simulink model "MASH"  (R2013b)
settings: Solver=FixedStepDiscrete  StartTime=0.0  StopTime=1.0  RelTol=1e-3
values from neighbouring files (symbols this model uses):
  ftest = 9e6    (= 9000000)    [Model.m]
  nLev = 512    [Model.m]
  Ts = 1/Fs    (= 2.03450520833e-09)    [Model.m]
libraries: dspsrcs4 x1
settings Model: Creator=o_cotte  LastModifiedBy=o_cotte
settings DataIOCC: LimitDataPoints=off  SaveFormat=Dataset
settings OptimizationCC: LifeSpan=auto  SimCompilerOptimization=off
settings DebuggingCC: UnderspecifiedInitializationDetection=Simplified  MergeDetectMultiDrivingBlocksExec=error  SolverPrmCheckMsg=none  FcnCallInpInsideContextMsg=error  FrameProcessingCompatibilityMsg=error  SFUnexpectedBacktrackingDiag=error  SFNoUnconditionalDefaultTransitionDiag=error
settings HardwareCC: ProdBitPerPointer=64  ProdLargestAtomicFloat=Float  ProdIntDivRoundTo=Zero  ProdEndianess=LittleEndian  ProdWordSize=64  ProdHWDeviceType=Intel->x86-64 (Windows64)
settings ModelReferenceCC: PropagateSignalLabelsOutOfModel=on
settings RTWCC: RTWCompilerOptimization=off
settings GRTTargetCC: CodeReplacementLibrary=None  GeneratePreprocessorConditionals=Use local settings  CPPClassGenCompliant=on

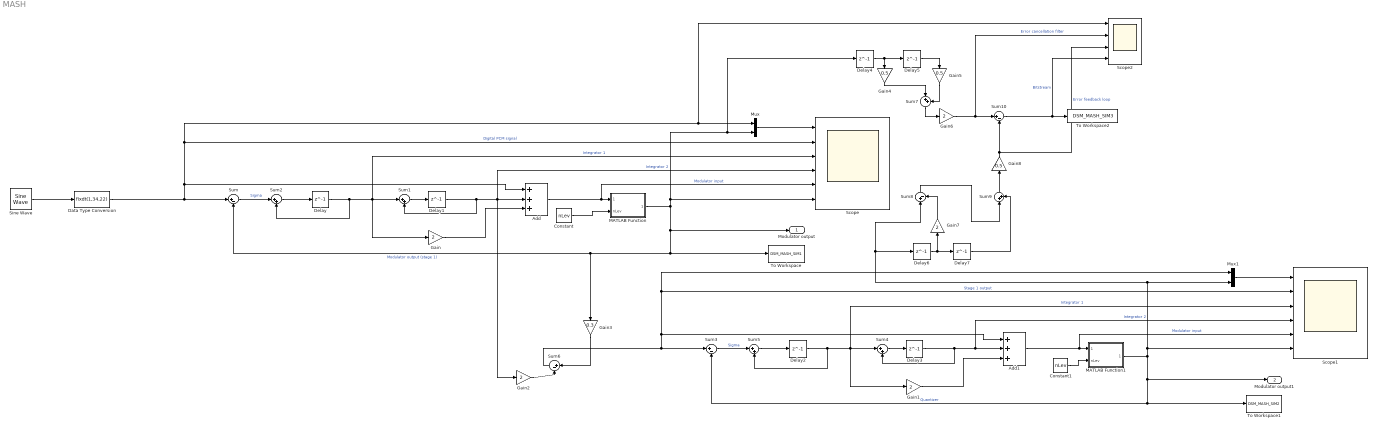
== system MASH ==
  Add : Sum  Inputs=+++  OutDataTypeStr=Inherit: Same as accumulator  LockScale=on
  Add1 : Sum  Inputs=+++  OutDataTypeStr=fixdt(1,34,23)
  Constant : Constant  Value=nLev
  Constant1 : Constant  Value=nLev
  Data Type Conversion : DataTypeConversion  OutDataTypeStr=fixdt(1,34,22)  LockScale=on
  Delay{,1..7} (8 alike) : Delay  DelayLength=1  InitialCondition=0
  Gain : Gain  Gain=2  OutDataTypeStr=Inherit: Same as input  LockScale=on
  Gain1 : Gain  Gain=2  OutDataTypeStr=fixdt(1,34,23)
  Gain2 : Gain  Gain=2  OutDataTypeStr=fixdt(1,34,23)
  Gain3 : Gain  Gain=0.3  OutDataTypeStr=Inherit: Same as input  LockScale=on
  Gain4 : Gain  Gain=0.5  OutDataTypeStr=Inherit: Same as input  ParamDataTypeStr=Inherit: Same as input  LockScale=on
  Gain5 : Gain  Gain=0.5  OutDataTypeStr=Inherit: Same as input  ParamDataTypeStr=Inherit: Same as input  LockScale=on
  Gain6 : Gain  Gain=2  OutDataTypeStr=Inherit: Same as input  LockScale=on
  Gain7 : Gain  Gain=2  OutDataTypeStr=fixdt(1,34,23)
  Gain8 : Gain  Gain=0.5  OutDataTypeStr=Inherit: Same as input  ParamDataTypeStr=Inherit: Same as input  LockScale=on
  MATLAB Function : MATLAB Function  TreatAsAtomicUnit=on
  MATLAB Function1 : MATLAB Function  TreatAsAtomicUnit=on
  Mux : Mux  Inputs=2
  Mux1 : Mux  Inputs=2
  Scope : Scope  NumInputPorts=6
  Scope1 : Scope  NumInputPorts=6
  Scope2 : Scope  NumInputPorts=4
  Sine Wave : dspsrcs4/Sine Wave  Amplitude=1  Frequency=ftest  Phase=0  SampleMode=Discrete  OutComplex=Real  CompMethod=Trigonometric fcn  TableSize=Speed  SampleTime=Ts  SamplesPerFrame=1  ResetState=Restart at time zero  dataType=double  wordLen=16  udDataType=sfix(16)  fracBitsMode=Best precision  numFracBits=15  OutDataTypeStr=double  LastOutDataTypeStr=double
  Sum{,3,6,8,10} (5 alike) : Sum  Inputs=|+-  OutDataTypeStr=Inherit: Same as accumulator  LockScale=on
  Sum{1..2,7,9} (4 alike) : Sum  Inputs=|++  OutDataTypeStr=Inherit: Same as accumulator  LockScale=on
  Sum4 : Sum  Inputs=|++  OutDataTypeStr=fixdt(1,34,23)
  Sum5 : Sum  Inputs=|++  OutDataTypeStr=fixdt(1,34,23)
  To Workspace : ToWorkspace  VariableName=DSM_MASH_SIM1  SampleTime=-1
  To Workspace1 : ToWorkspace  VariableName=DSM_MASH_SIM2  SampleTime=-1
  To Workspace2 : ToWorkspace  VariableName=DSM_MASH_SIM3  SampleTime=-1
  Modulator output : Outport
  Modulator output1 : Outport  Port=2
  wires:
  Gain5/1 -> Sum7/2
  Gain/1 -> Add/3
  Delay2/1 -> Sum5/2, Sum4/1, Scope1/3, Gain1/1  "Integrator 1"
  Mux/1 -> Scope/1
  Delay7/1 -> Sum9/2
  Delay1/1 -> Sum1/2, Gain2/1, Scope/4, Add/2  "Integrator 2"
  Sum3/1 -> Sum5/1  "Sigma"
  Delay5/1 -> Gain5/1
  Mux1/1 -> Scope1/1
  Add1/1 -> MATLAB Function1/1(quant_in), Scope1/5  "Modulator input"
  MATLAB Function1/1(quant_out) -> Scope1/6, Sum8/1, Delay6/1, Mux1/2, Modulator output1/1, Sum3/2, To Workspace1/1  "Quantizer"
  Gain7/1 -> Sum8/2
  Delay4/1 -> Delay5/1, Gain4/1
  Sum9/1 -> Gain8/1
  Constant/1 -> MATLAB Function/2(nLev)
  Data Type Conversion/1 -> Sum/1, Scope/2, Scope2/1, Mux/1, Add/1  "Digital PCM signal"
  Sum4/1 -> Delay3/1
  Add/1 -> Scope/5, MATLAB Function/1(quant_in)  "Modulator input"
  Sum6/1 -> Sum3/1, Scope1/2, Mux1/1, Add1/1  "Stage 1 output"
  Sum2/1 -> Delay/1
  Sum/1 -> Sum2/1  "Sigma"
  Gain3/1 -> Sum6/1
  Delay/1 -> Sum2/2, Sum1/1, Scope/3, Gain/1  "Integrator 1"
  Gain6/1 -> Sum10/1, Scope2/2  "Error cancellation filter"
  Gain2/1 -> Sum6/2
  Sum8/1 -> Sum9/1
  Gain1/1 -> Add1/3
  Sum10/1 -> Scope2/4, To Workspace2/1  "Bitstream"
  Sine Wave/1 -> Data Type Conversion/1
  Delay6/1 -> Gain7/1, Delay7/1
  Constant1/1 -> MATLAB Function1/2(nLev)
  Delay3/1 -> Sum4/2, Scope1/4, Add1/2  "Integrator 2"
  Gain4/1 -> Sum7/1
  Sum7/1 -> Gain6/1
  Sum5/1 -> Delay2/1
  Gain8/1 -> Scope2/3, Sum10/2  "Error feedback loop"
  MATLAB Function/1(quant_out) -> Scope/6, Delay4/1, Mux/2, Modulator output/1, Gain3/1, Sum/2, To Workspace/1  "Modulator output (stage 1)"
  Sum1/1 -> Delay1/1

== matlab function MASH/MATLAB Function ==
  data: quant_in input; quant_out output; nLev input
function quant_out = fcn(quant_in,nLev)
%#codegen
% if u < 0
%     y = fi(-1,1,34,23);
% else
%     y = fi(1,1,34,23);
% end
% nLev=512;
st=fi(nLev-2,1,34,22);
quant_out=fi(0,1,34,22);
if quant_in < -st
    quant_out = fi(-nLev+1,1,34,22);
    %     return;
elseif quant_in >= st
    quant_out = fi(nLev-1,1,34,22);
    %     return;
else
    for n=1:nLev-2
        k=fi(n,1,34,22);
        if quant_in >= -nLev + 2*k && quant_in < -nLev + 2*(k+1)
            quant_out = fi(2*k-1-nLev,1,34,22);
        end
    end
end

== matlab function MASH/MATLAB Function1 ==
  data: quant_in input; quant_out output; nLev input
function quant_out = fcn(quant_in,nLev)
%#codegen
% if u < 0
%     y = fi(-1,1,34,23);
% else
%     y = fi(1,1,34,23);
% end
% nLev=512;
st=fi(nLev-2,1,34,22);
quant_out=fi(0,1,34,22);
if quant_in < -st
    quant_out = fi(-nLev+1,1,34,22);
    %     return;
elseif quant_in >= st
    quant_out = fi(nLev-1,1,34,22);
    %     return;
else
    for n=1:nLev-2
        k=fi(n,1,34,22);
        if quant_in >= -nLev + 2*k && quant_in < -nLev + 2*(k+1)
            quant_out = fi(2*k-1-nLev,1,34,22);
        end
    end
end

== matlab function MASH/MATLAB Function1 ==
  data: quant_in input; quant_out output; nLev input
function quant_out = fcn(quant_in,nLev)
%#codegen
st=fi(nLev-2,1,34,22);
quant_out=fi(0,1,34,22);
if quant_in < -st
    quant_out = fi(-nLev+1,1,34,22);
    %     return;
elseif quant_in >= st
    quant_out = fi(nLev-1,1,34,22);
    %     return;
else
    for n=1:nLev-2
        k=fi(n,1,34,22);
        if quant_in >= -nLev + 2*k && quant_in < -nLev + 2*(k+1)
            quant_out = fi(2*k-1-nLev,1,34,22);
        end
    end
end

== matlab function MASH/MATLAB Function ==
  data: quant_in input; quant_out output; nLev input
function quant_out = fcn(quant_in,nLev)
%#codegen
st=fi(nLev-2,1,34,22);
quant_out=fi(0,1,34,22);
if quant_in < -st
    quant_out = fi(-nLev+1,1,34,22);
    %     return;
elseif quant_in >= st
    quant_out = fi(nLev-1,1,34,22);
    %     return;
else
    for n=1:nLev-2
        k=fi(n,1,34,22);
        if quant_in >= -nLev + 2*k && quant_in < -nLev + 2*(k+1)
            quant_out = fi(2*k-1-nLev,1,34,22);
        end
    end
end
